simulink model "Enable_trigger_subsystem"  (R2020b)
settings: Solver=VariableStepAuto  StartTime=0.0  StopTime=5  FixedStep=1  RelTol=1e-3
libraries: simulink x1
settings Model: Creator=Training  LastModifiedBy=Training

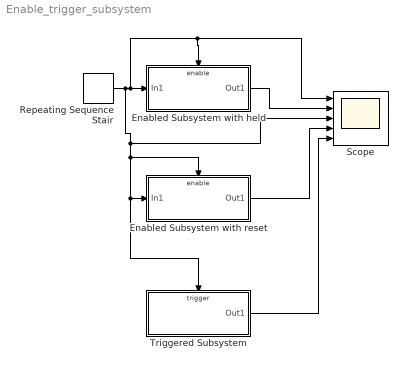
== system Enable_trigger_subsystem ==
  Enabled Subsystem with held : Subsystem  TreatAsAtomicUnit=on
  Enabled Subsystem with reset : Subsystem  TreatAsAtomicUnit=on
  Repeating Sequence Stair : simulink/Sources/Repeating Sequence Stair  OutValues=[0 0 0 1 1 0 1].'  tsamp=-1  OutMin=[]  OutMax=[]  OutDataTypeStr=double  OutputDataTypeScalingMode=double  OutDataType=fixdt(0,8)  ConRadixGroup=Best Precision: Vector-wise  OutScaling=2^-12
  Scope : Scope  NumInputPorts=5
  Triggered Subsystem : Subsystem  TreatAsAtomicUnit=on
  wires:
  Repeating Sequence Stair/1 -> Enabled Subsystem with reset/Enable, Triggered Subsystem/Trigger, Enabled Subsystem with reset/1(In1), Scope/3, Scope/1, Enabled Subsystem with held/Enable, Enabled Subsystem with held/1(In1)
  Enabled Subsystem with held/1(Out1) -> Scope/2
  Enabled Subsystem with reset/1(Out1) -> Scope/4
  Triggered Subsystem/1(Out1) -> Scope/5

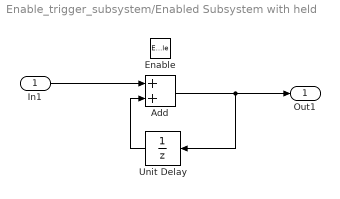
== system Enable_trigger_subsystem/Enabled Subsystem with held ==
  In1 : Inport
  Enable : EnablePort
  Add : Sum
  Unit Delay : UnitDelay  SampleTime=-1  HasFrameUpgradeWarning=on
  Out1 : Outport
  wires:
  In1/1 -> Add/1
  Unit Delay/1 -> Add/2
  Add/1 -> Out1/1, Unit Delay/1

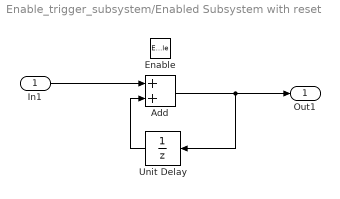
== system Enable_trigger_subsystem/Enabled Subsystem with reset ==
  In1 : Inport
  Enable : EnablePort  StatesWhenEnabling=reset
  Add : Sum
  Unit Delay : UnitDelay  SampleTime=-1  HasFrameUpgradeWarning=on
  Out1 : Outport
  wires:
  In1/1 -> Add/1
  Unit Delay/1 -> Add/2
  Add/1 -> Out1/1, Unit Delay/1

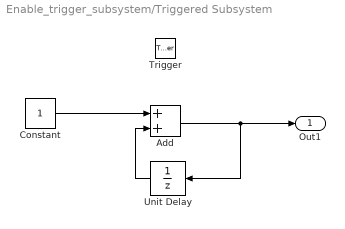
== system Enable_trigger_subsystem/Triggered Subsystem ==
  Trigger : TriggerPort  TriggerType=either  VariantControl=Variant
  Add : Sum
  Constant : Constant
  Unit Delay : UnitDelay  SampleTime=-1  HasFrameUpgradeWarning=on
  Out1 : Outport
  wires:
  Unit Delay/1 -> Add/2
  Constant/1 -> Add/1
  Add/1 -> Out1/1, Unit Delay/1
